simulink model "MLI_MODEL"  (R2024b)
settings: Solver=VariableStepAuto  StartTime=0.0  StopTime=10.0  RelTol=1e-3
libraries: spsMosfetLib x8, simulink x4, spsSeriesRLCBranchLib x3, spsRMSLib x2, spsDCVoltageSourceLib x2, spsGroundLib x2, spsTHDLib x2, spsCurrentMeasurementLib x1, spsVoltageMeasurementLib x1, spspowerguiLib x1
settings Model: Creator=evadi  LastModifiedBy=hp
settings SolverCC: ZeroCrossAlgorithm=Adaptive
settings DebuggingCC: IgnoredZcDiagnostic=none

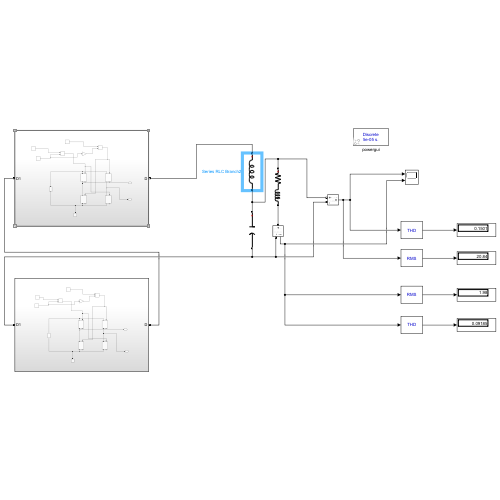
[thumbnail: Simulink's stored preview of the top-level diagram]
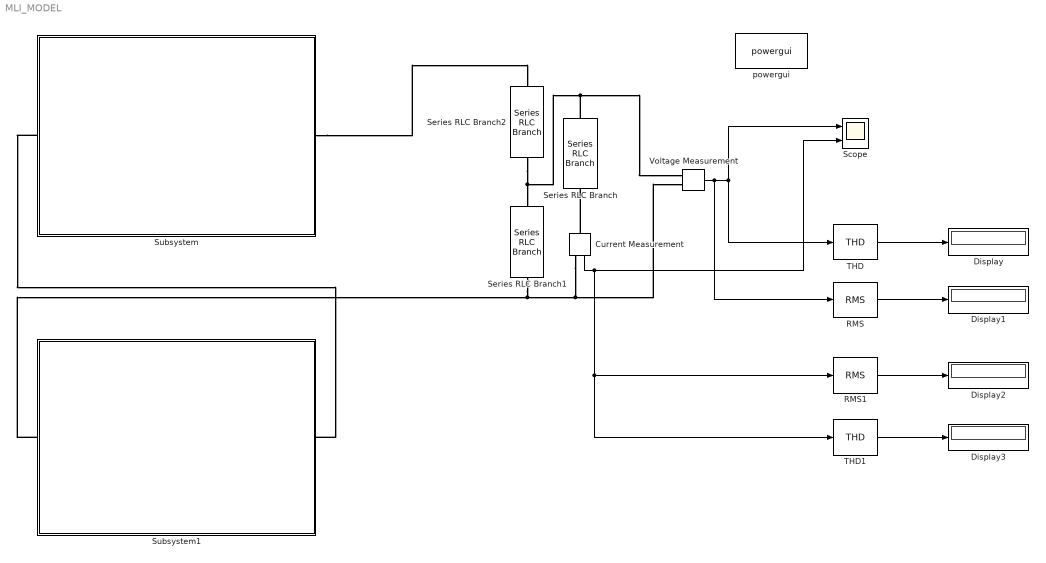
== system MLI_MODEL ==
  Current Measurement : spsCurrentMeasurementLib/Current Measurement  PhasorSimulation=off  OutputType=Complex  PSBequivalent=0
  Display{,1..3} (4 alike) : Display
  RMS : spsRMSLib/RMS  TrueRMS=on  Freq=50  RMSInit=0  Ts=0
  RMS1 : spsRMSLib/RMS  TrueRMS=on  Freq=50  RMSInit=0  Ts=0
  Scope : Scope  NumInputPorts=2
  Series RLC Branch : spsSeriesRLCBranchLib/Series RLC Branch  LConnTagsString=__new0  RConnTagsString=__new0  BranchType=RL  Resistance=10  Inductance=10e-3  SetiL0=off  InitialCurrent=0  Capacitance=1e-6  Setx0=off  InitialVoltage=0  Measurements=None
  Series RLC Branch1 : spsSeriesRLCBranchLib/Series RLC Branch  LConnTagsString=__new0  RConnTagsString=__new0  BranchType=C  Resistance=10  Inductance=40e-3  SetiL0=off  InitialCurrent=0  Capacitance=33e-6  Setx0=off  InitialVoltage=0  Measurements=None
  Series RLC Branch2 : spsSeriesRLCBranchLib/Series RLC Branch  LConnTagsString=__new0  RConnTagsString=__new0  BranchType=L  Resistance=10  Inductance=70e-3  SetiL0=off  InitialCurrent=0  Capacitance=25e-6  Setx0=off  InitialVoltage=0  Measurements=None
  Subsystem : Subsystem
  Subsystem1 : Subsystem
  THD : spsTHDLib/THD  Freq=50  Ts=0
  THD1 : spsTHDLib/THD  Freq=50  Ts=0
  Voltage Measurement : spsVoltageMeasurementLib/Voltage Measurement  PhasorSimulation=off  OutputType=Complex  PSBequivalent=0
  powergui : spspowerguiLib/powergui  Priority=1  SimulationMode=Discrete  SampleTime=50e-6  frequency=60  Iterations=50  frequencyindice=0  Pbase=100e6  ErrMax=1e-4  UnitsV=kV  UnitsW=MW  buscounter=0  FunctionMessages=off  echomessages=off  EnableUseOfTLC=off  CurrentSourceSwitches=off  DisableSnubberDevices=off  DisableRonSwitches=off  DisableVfSwitches=off  DisplayEquations=off  AutomaticDiscreteSolvers=off  SolverType=Tustin/Backward Euler (TBE)  Interpol=off  ExternalGateDelay=off  methode=off  Ts=100  x0status=blocks  SPID=on  SwTol=0  HookPort=off  NonlinearTolerance=1e-4  nMaxIteration=100  ContinueOnMaxIteration=off  RestoreLinks=warning  ResistiveCurrentMeasurement=off  Frange=[0:2:500]  Ylog=off  Xlog=on  ShowGrid=off  save=off  variable=ZData  structure=0  ZoomFFT=off  StartTime=0.0  cycles=1  DisplayStyle=1  fundamental=60  FreqAxis=off  MaxFrequency=1000  frequencyindicesteady=1  RmsSteady=1  display=off
  wires:
  THD1/1 -> Display3/1
  THD/1 -> Display/1
  RMS1/1 -> Display2/1
  Voltage Measurement/1 -> RMS/1, Scope/1, THD/1
  Current Measurement/1 -> RMS1/1, THD1/1, Scope/2
  RMS/1 -> Display1/1
  connections:
  Subsystem/LConn1 -- Subsystem1/RConn1
  Subsystem1/LConn1 -- Series RLC Branch1/RConn1 -- Current Measurement/RConn1 -- Voltage Measurement/LConn2
  Current Measurement/LConn1 -- Series RLC Branch/RConn1
  Series RLC Branch2/RConn1 -- Voltage Measurement/LConn1 -- Series RLC Branch/LConn1 -- Series RLC Branch1/LConn1
  Subsystem/RConn1 -- Series RLC Branch2/LConn1

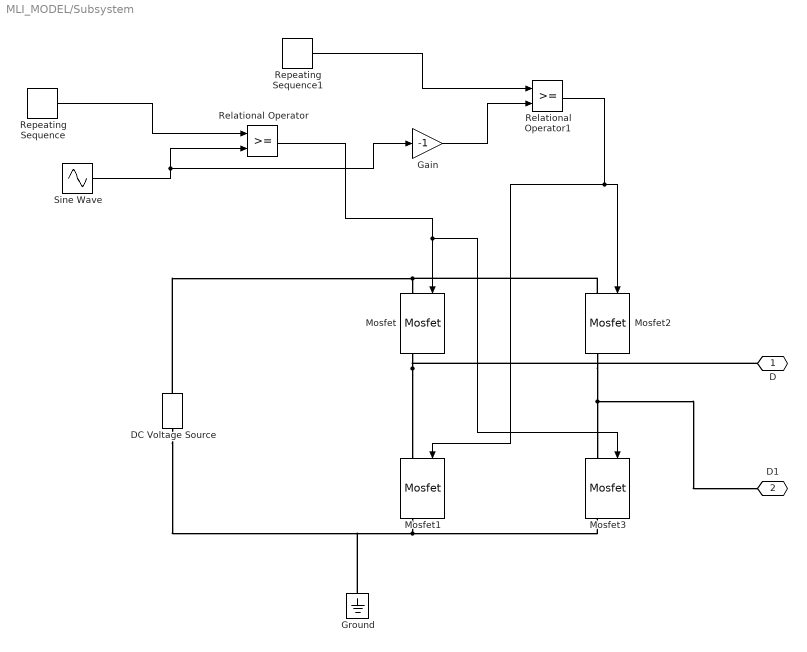
== system MLI_MODEL/Subsystem ==
  DC Voltage Source : spsDCVoltageSourceLib/DC Voltage Source  Amplitude=100  Measurements=None
  Gain : Gain  Gain=-1
  Ground : spsGroundLib/Ground  LConnTagsString=a
  Mosfet{,1..3} (4 alike) : spsMosfetLib/Mosfet  Ron=0.1  Lon=0  Rd=0.01  Vfd=0  IC=0  Rs=1e5  Cs=inf  Measurements=on
  Relational Operator : RelationalOperator  OutDataTypeStr=boolean  RndMeth=Simplest  InputSameDT=off
  Relational Operator1 : RelationalOperator  OutDataTypeStr=boolean  RndMeth=Simplest  InputSameDT=off
  Repeating Sequence : simulink/Sources/Repeating Sequence  rep_seq_t=[0 1]  rep_seq_y=[0 1]
  Repeating Sequence1 : simulink/Sources/Repeating Sequence  rep_seq_t=[0 1]  rep_seq_y=[0.1 0.9]
  Sine Wave : Sin  Amplitude=2  Frequency=2*pi*50  SampleTime=0
  D : PMIOPort  Side=Right
  D1 : PMIOPort  Port=2  Side=Left
  wires:
  Relational Operator1/1 -> Mosfet1/1, Mosfet2/1
  Repeating Sequence/1 -> Relational Operator/1
  Gain/1 -> Relational Operator1/2
  Repeating Sequence1/1 -> Relational Operator1/1
  Relational Operator/1 -> Mosfet3/1, Mosfet/1
  Sine Wave/1 -> Gain/1, Relational Operator/2
  connections:
  Mosfet1/RConn1 -- Ground/LConn1 -- DC Voltage Source/LConn1 -- Mosfet3/RConn1
  DC Voltage Source/RConn1 -- Mosfet2/LConn1 -- Mosfet/LConn1
  Mosfet/RConn1 -- Mosfet1/LConn1 -- D/RConn1
  Mosfet2/RConn1 -- D1/RConn1 -- Mosfet3/LConn1

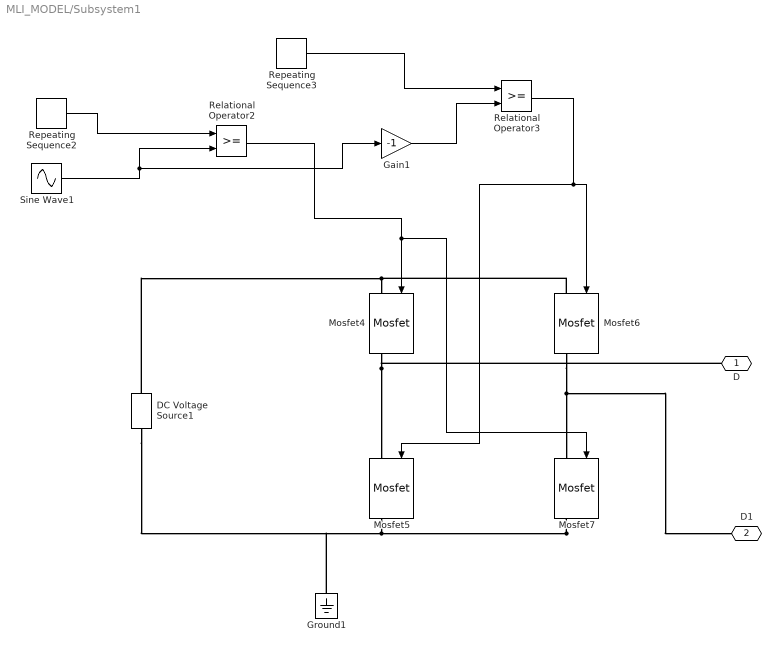
== system MLI_MODEL/Subsystem1 ==
  DC Voltage Source1 : spsDCVoltageSourceLib/DC Voltage Source  Amplitude=100  Measurements=None
  Gain1 : Gain  Gain=-1
  Ground1 : spsGroundLib/Ground  LConnTagsString=a
  Mosfet{4..7} (4 alike) : spsMosfetLib/Mosfet  Ron=0.1  Lon=0  Rd=0.01  Vfd=0  IC=0  Rs=1e5  Cs=inf  Measurements=on
  Relational Operator2 : RelationalOperator  OutDataTypeStr=boolean  RndMeth=Simplest  InputSameDT=off
  Relational Operator3 : RelationalOperator  OutDataTypeStr=boolean  RndMeth=Simplest  InputSameDT=off
  Repeating Sequence2 : simulink/Sources/Repeating Sequence  rep_seq_t=[0 1]  rep_seq_y=[1 2]
  Repeating Sequence3 : simulink/Sources/Repeating Sequence  rep_seq_t=[0 1]  rep_seq_y=[1.1 1.9]
  Sine Wave1 : Sin  Amplitude=2  Frequency=2*pi*50  SampleTime=0
  D : PMIOPort  Side=Right
  D1 : PMIOPort  Port=2  Side=Left
  wires:
  Sine Wave1/1 -> Gain1/1, Relational Operator2/2
  Relational Operator2/1 -> Mosfet7/1, Mosfet4/1
  Gain1/1 -> Relational Operator3/2
  Repeating Sequence2/1 -> Relational Operator2/1
  Relational Operator3/1 -> Mosfet5/1, Mosfet6/1
  Repeating Sequence3/1 -> Relational Operator3/1
  connections:
  Mosfet7/RConn1 -- Ground1/LConn1 -- DC Voltage Source1/LConn1 -- Mosfet5/RConn1
  Mosfet4/LConn1 -- DC Voltage Source1/RConn1 -- Mosfet6/LConn1
  Mosfet6/RConn1 -- Mosfet7/LConn1 -- D1/RConn1
  Mosfet4/RConn1 -- Mosfet5/LConn1 -- D/RConn1
